simulink model "uz_ssi_interface_2023a"  (R2023a)
settings: Solver=FixedStepDiscrete  StartTime=0.0  StopTime=0.003  RelTol=1e-3
values from neighbouring files (symbols this model uses):
  binary_or_gray = false    [uz_ssi_interface_init.m]
  bit_sum = ssi_encoder_bit_width_multi_turn+ssi_encoder_bit_width_single_turn+ssi_encoder_number_of_status_bits    [uz_ssi_interface_init.m]
  delay_first_clk_on_off = true    [uz_ssi_interface_init.m]
  f_ADC = 10e3    (= 10000)    [uz_ssi_interface_init.m]
  f_clock = 100e6    (= 100000000)    [uz_ssi_interface_init.m]
  ssi_clk_divider = 25    [uz_ssi_interface_init.m]
  ssi_encoder_bit_width_multi_turn = uint32(0)    [uz_ssi_interface_init.m]
  ssi_encoder_bit_width_single_turn = uint32(14)    [uz_ssi_interface_init.m]
  ssi_encoder_number_of_status_bits = uint32(0)    [uz_ssi_interface_init.m]
  t_ADC = 1/f_ADC    (= 0.0001)    [uz_ssi_interface_init.m]
  t_clock = 1/f_clock    (= 1e-08)    [uz_ssi_interface_init.m]
undefined symbols (not defined in the file or in its folder): PLL
libraries: hdlsllib x42, simulink x14, simulink_extras x5, spsSampleandHoldLib x1
(part 1 of 2)
settings Model: DataTypeOverride=Off  Creator=micha  LastModifiedBy=micha
settings SolverCC: AlgebraicLoopSolver=TrustRegion
settings DataIOCC: LimitDataPoints=on  SaveOutput=off  SaveTime=off
settings OptimizationCC: BlockReduction=off  ConditionallyExecuteInputs=off  DefaultParameterBehavior=Inlined  LifeSpan=inf
settings DebuggingCC: AlgebraicLoopMsg=error  SingleTaskRateTransMsg=error  UnconnectedInputMsg=warning  UnconnectedOutputMsg=warning  UnconnectedLineMsg=warning  AllowSymbolicDim=off  StrictBusMsg=ErrorOnBusTreatedAsVector  SFUnexpectedBacktrackingDiag=warning  SFNoUnconditionalDefaultTransitionDiag=warning  SFExecutionAtInitializationDiag=none  ArithmeticOperatorsInVariantConditions=warning
settings HardwareCC: ProdBitPerPointer=32  ProdBitPerSizeT=32  ProdBitPerPtrDiffT=32  ProdLargestAtomicFloat=None  ProdIntDivRoundTo=Undefined  ProdEndianess=Unspecified  ProdWordSize=32  ProdHWDeviceType=ASIC/FPGA->ASIC/FPGA  ProdEqTarget=off
settings ModelReferenceCC: EnableRefExpFcnMdlSchedulingChecks=on
settings SFSimCC: SimUseLocalCustomCode=off  CustomCodeUndefinedFunction=UseInterfaceOnly
settings RTWCC: RTWUseLocalCustomCode=off  DLArmComputeVersion=19.05
settings CodeAppCC: StateflowObjectComments=on
settings GRTTargetCC: TargetLangStandard=C89/C90 (ANSI)
settings ConfigComp: CovScope=ReferencedModels  CovMetricSettings=dw  CovSaveCumulativeToWorkspaceVar=on  CovSaveSingleToWorkspaceVar=on  CovExternalEMLEnable=off  CovSFcnEnable=off

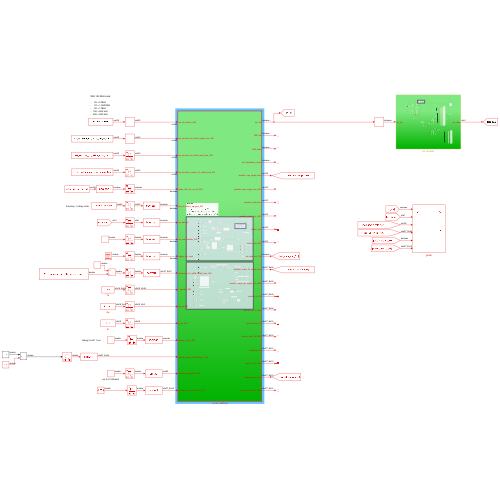
[thumbnail: Simulink's stored preview of the top-level diagram]
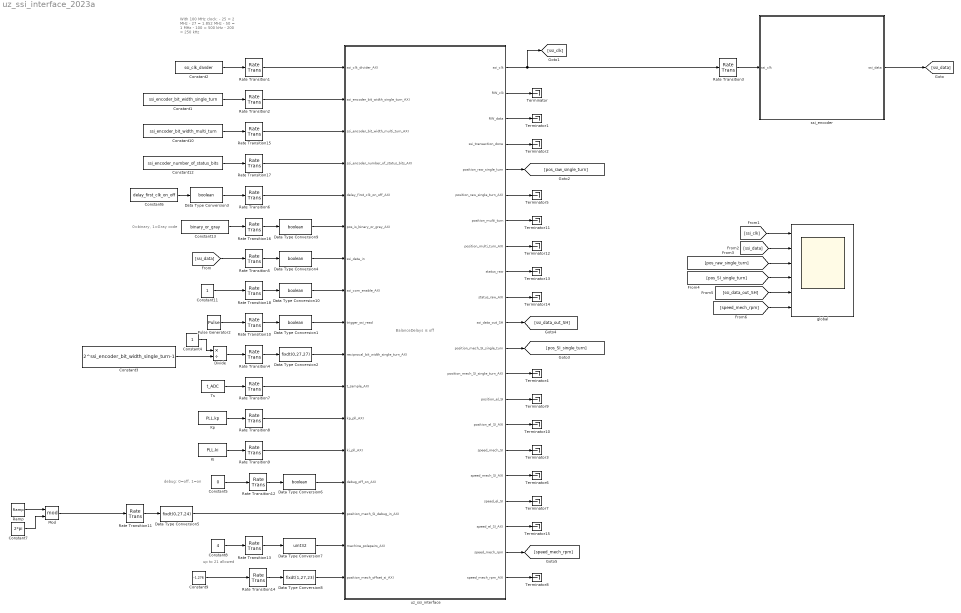
== system uz_ssi_interface_2023a ==
  note: up to 21 allowed
  note: debug: 0=off, 1=on
  note: BalanceDelays is off
  note: With 100 MHz clock:
      |
      | -     25 = 2 MHz
      | -     27 = 1.852 MHz
      | -     50 = 1 MHz
      | -   100 = 500 kHz
      | -   200 = 250 kHz
  note: 0=binary, 1=Gray code
  Constant1 : Constant  Value=ssi_encoder_bit_width_single_turn  OutDataTypeStr=uint32  SampleTime=t_clock
  Constant10 : Constant  Value=ssi_encoder_bit_width_multi_turn  OutDataTypeStr=uint32  SampleTime=t_clock
  Constant11 : Constant  SampleTime=t_clock
  Constant12 : Constant  Value=ssi_encoder_number_of_status_bits  OutDataTypeStr=uint32  SampleTime=t_clock
  Constant13 : Constant  Value=binary_or_gray  OutDataTypeStr=uint32  SampleTime=t_clock
  Constant2 : Constant  Value=ssi_clk_divider  OutDataTypeStr=uint32  SampleTime=t_clock
  Constant3 : Constant  Value=2^ssi_encoder_bit_width_single_turn-1  OutDataTypeStr=double  SampleTime=t_clock
  Constant4 : Constant  SampleTime=t_clock
  Constant5 : Constant  Value=0  SampleTime=t_clock
  Constant6 : Constant  Value=delay_first_clk_on_off  OutDataTypeStr=uint32  SampleTime=t_clock
  Constant7 : Constant  Value=2*pi  SampleTime=t_clock
  Constant8 : Constant  Value=4  SampleTime=t_clock
  Constant9 : Constant  Value=-1.276  SampleTime=t_clock
  Data Type Conversion{1,3..4,6,9..10} (6 alike) : DataTypeConversion  OutDataTypeStr=boolean  SaturateOnIntegerOverflow=off  RndMeth=Floor
  Data Type Conversion2 : DataTypeConversion  OutDataTypeStr=fixdt(0,27,27)  SaturateOnIntegerOverflow=off  RndMeth=Floor
  Data Type Conversion5 : DataTypeConversion  OutDataTypeStr=fixdt(0,27,24)  SaturateOnIntegerOverflow=off  RndMeth=Floor
  Data Type Conversion7 : DataTypeConversion  OutDataTypeStr=uint32  SaturateOnIntegerOverflow=off  RndMeth=Floor
  Data Type Conversion8 : DataTypeConversion  OutDataTypeStr=fixdt(1,27,23)  SaturateOnIntegerOverflow=off  RndMeth=Floor
  Divide : Product  Inputs=*/
  Ki : Constant  Value=PLL.ki  OutDataTypeStr=fixdt(0,18,0)  SampleTime=-1
  Kp : Constant  Value=PLL.kp  OutDataTypeStr=fixdt(0,18,5)  SampleTime=-1
  Mod : Math  Operator=mod
  Pulse Generator2 : DiscretePulseGenerator  Period=f_clock/f_ADC  PulseWidth=0.04*f_clock/f_ADC  SampleTime=t_clock
  Ramp : simulink/Sources/Ramp  slope=2*pi*100  start=7.5e-5  InitialOutput=0
  Rate Transition{1..18} (18 alike) : RateTransition  OutPortSampleTime=t_clock
  Terminator{,1..15} (16 alike) : Terminator
  Ts : Constant  Value=t_ADC  OutDataTypeStr=fixdt(0,18,24)  SampleTime=-1
  global : Scope  NumInputPorts=6
  ssi_encoder : Subsystem
  uz_ssi_interface : Subsystem  TreatAsAtomicUnit=on
  wires:
  Rate Transition10/1 -> Data Type Conversion1/1
  Pulse Generator2/1 -> Rate Transition10/1
  Constant2/1 -> Rate Transition1/1
  Rate Transition1/1 -> uz_ssi_interface/1(ssi_clk_divider_AXI)
  Constant1/1 -> Rate Transition2/1
  Rate Transition2/1 -> uz_ssi_interface/2(ssi_encoder_bit_width_single_turn_AXI)
  Rate Transition3/1 -> ssi_encoder/1(ssi_clk)
  ssi_encoder/1(ssi_data) -> [ssi_data]
  [ssi_data] -> Rate Transition5/1
  uz_ssi_interface/1(ssi_clk) -> [ssi_clk], Rate Transition3/1
  uz_ssi_interface/3(RW_data) -> Terminator1/1
  uz_ssi_interface/4(ssi_transaction_done) -> Terminator2/1
  uz_ssi_interface/2(RW_clk) -> Terminator/1
  Data Type Conversion1/1 -> uz_ssi_interface/9(trigger_ssi_read)
  Rate Transition6/1 -> uz_ssi_interface/5(delay_first_clk_on_off_AXI)
  Data Type Conversion3/1 -> Rate Transition6/1
  Constant6/1 -> Data Type Conversion3/1
  uz_ssi_interface/6(position_raw_single_turn_AXI) -> Terminator5/1
  Rate Transition5/1 -> Data Type Conversion4/1
  Data Type Conversion4/1 -> uz_ssi_interface/7(ssi_data_in)
  Constant3/1 -> Divide/2
  Rate Transition4/1 -> Data Type Conversion2/1
  Data Type Conversion2/1 -> uz_ssi_interface/10(reciprocal_bit_width_single_turn_AXI)
  Constant4/1 -> Divide/1
  Divide/1 -> Rate Transition4/1
  uz_ssi_interface/13(position_mech_SI_single_turn_AXI) -> Terminator4/1
  Ts/1 -> Rate Transition7/1
  Rate Transition7/1 -> uz_ssi_interface/11(t_sample_AXI)
  Kp/1 -> Rate Transition8/1
  Rate Transition8/1 -> uz_ssi_interface/12(kp_pll_AXI)
  Ki/1 -> Rate Transition9/1
  Rate Transition9/1 -> uz_ssi_interface/13(ki_pll_AXI)
  uz_ssi_interface/16(speed_mech_SI) -> Terminator3/1
  uz_ssi_interface/17(speed_mech_SI_AXI) -> Terminator6/1
  Rate Transition11/1 -> Data Type Conversion5/1
  Data Type Conversion5/1 -> uz_ssi_interface/15(position_mech_SI_debug_in_AXI)
  Data Type Conversion6/1 -> uz_ssi_interface/14(debug_off_on_AXI)
  Rate Transition12/1 -> Data Type Conversion6/1
  Constant5/1 -> Rate Transition12/1
  Mod/1 -> Rate Transition11/1
  Ramp/1 -> Mod/1
  Constant7/1 -> Mod/2
  uz_ssi_interface/21(speed_mech_rpm_AXI) -> Terminator8/1
  Rate Transition13/1 -> Data Type Conversion7/1
  Data Type Conversion7/1 -> uz_ssi_interface/16(machine_polepairs_AXI)
  Constant8/1 -> Rate Transition13/1
  Rate Transition14/1 -> Data Type Conversion8/1
  Constant9/1 -> Rate Transition14/1
  Data Type Conversion8/1 -> uz_ssi_interface/17(position_mech_offset_si_AXI)
  uz_ssi_interface/14(position_el_SI) -> Terminator9/1
  uz_ssi_interface/15(position_el_SI_AXI) -> Terminator10/1
  Rate Transition15/1 -> uz_ssi_interface/3(ssi_encoder_bit_width_multi_turn_AXI)
  Constant10/1 -> Rate Transition15/1
  Rate Transition16/1 -> Data Type Conversion9/1
  Constant13/1 -> Rate Transition16/1
  Data Type Conversion9/1 -> uz_ssi_interface/6(pos_is_binary_or_gray_AXI)
  Rate Transition17/1 -> uz_ssi_interface/4(ssi_encoder_number_of_status_bits_AXI)
  Constant12/1 -> Rate Transition17/1
  Data Type Conversion10/1 -> uz_ssi_interface/8(ssi_com_enable_AXI)
  Rate Transition18/1 -> Data Type Conversion10/1
  Constant11/1 -> Rate Transition18/1
  uz_ssi_interface/7(position_multi_turn) -> Terminator11/1
  uz_ssi_interface/8(position_multi_turn_AXI) -> Terminator12/1
  uz_ssi_interface/9(status_raw) -> Terminator13/1
  uz_ssi_interface/10(status_raw_AXI) -> Terminator14/1
  uz_ssi_interface/19(speed_el_SI_AXI) -> Terminator15/1
  uz_ssi_interface/18(speed_el_SI) -> Terminator7/1
  [ssi_clk] -> global/1
  [ssi_data] -> global/2
  uz_ssi_interface/5(position_raw_single_turn) -> [pos_raw_single_turn]
  [pos_raw_single_turn] -> global/3
  [pos_SI_single_turn] -> global/4
  uz_ssi_interface/12(position_mech_SI_single_turn) -> [pos_SI_single_turn]
  uz_ssi_interface/11(ssi_data_out_SH) -> [ssi_data_out_SH]
  [ssi_data_out_SH] -> global/5
  uz_ssi_interface/20(speed_mech_rpm) -> [speed_mech_rpm]
  [speed_mech_rpm] -> global/6

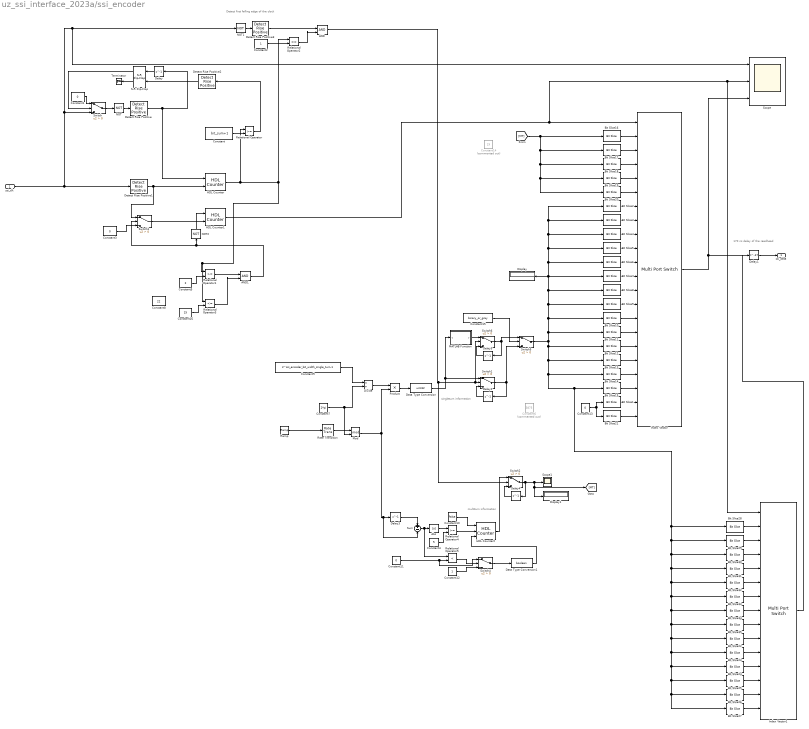
== system uz_ssi_interface_2023a/ssi_encoder ==
  note: multiturn information
  note: 170 ns delay of the readhead
  note: Detect first falling edge of the clock
  note: singleturn information
  ssi_clk : Inport
  AND : Logic  IconShape=distinctive  AllPortsSameDT=off  OutDataTypeStr=boolean
  AND1 : Logic  IconShape=distinctive  AllPortsSameDT=off  OutDataTypeStr=boolean
  Abs : Abs  SaturateOnIntegerOverflow=off
  Bit Slice{1,14,19,26} (4 alike) : hdlsllib/Logic and Bit Operations/Bit Slice  lidx=1  ridx=1
  Bit Slice10 : hdlsllib/Logic and Bit Operations/Bit Slice  lidx=5  ridx=5
  Bit Slice11 : hdlsllib/Logic and Bit Operations/Bit Slice  lidx=4  ridx=4
  Bit Slice12 : hdlsllib/Logic and Bit Operations/Bit Slice  lidx=3  ridx=3
  Bit Slice13 : hdlsllib/Logic and Bit Operations/Bit Slice  lidx=2  ridx=2
  Bit Slice{15,20..21,27} (4 alike) : hdlsllib/Logic and Bit Operations/Bit Slice  lidx=0  ridx=0
  Bit Slice16 : hdlsllib/Logic and Bit Operations/Bit Slice  lidx=4  ridx=4
  Bit Slice17 : hdlsllib/Logic and Bit Operations/Bit Slice  lidx=3  ridx=3
  Bit Slice18 : hdlsllib/Logic and Bit Operations/Bit Slice  lidx=2  ridx=2
  Bit Slice2 : hdlsllib/Logic and Bit Operations/Bit Slice  lidx=13  ridx=13
  Bit Slice22 : hdlsllib/Logic and Bit Operations/Bit Slice  lidx=5  ridx=5
  Bit Slice23 : hdlsllib/Logic and Bit Operations/Bit Slice  lidx=4  ridx=4
  Bit Slice24 : hdlsllib/Logic and Bit Operations/Bit Slice  lidx=3  ridx=3
  Bit Slice25 : hdlsllib/Logic and Bit Operations/Bit Slice  lidx=2  ridx=2
  Bit Slice28 : hdlsllib/Logic and Bit Operations/Bit Slice  lidx=13  ridx=13
  Bit Slice29 : hdlsllib/Logic and Bit Operations/Bit Slice  lidx=12  ridx=12
  Bit Slice3 : hdlsllib/Logic and Bit Operations/Bit Slice  lidx=12  ridx=12
  Bit Slice30 : hdlsllib/Logic and Bit Operations/Bit Slice  lidx=11  ridx=11
  Bit Slice31 : hdlsllib/Logic and Bit Operations/Bit Slice  lidx=10  ridx=10
  Bit Slice32 : hdlsllib/Logic and Bit Operations/Bit Slice  lidx=9  ridx=9
  Bit Slice33 : hdlsllib/Logic and Bit Operations/Bit Slice  lidx=8  ridx=8
  Bit Slice34 : hdlsllib/Logic and Bit Operations/Bit Slice  lidx=7  ridx=7
  Bit Slice35 : hdlsllib/Logic and Bit Operations/Bit Slice  lidx=6  ridx=6
  Bit Slice4 : hdlsllib/Logic and Bit Operations/Bit Slice  lidx=11  ridx=11
  Bit Slice5 : hdlsllib/Logic and Bit Operations/Bit Slice  lidx=10  ridx=10
  Bit Slice6 : hdlsllib/Logic and Bit Operations/Bit Slice  lidx=9  ridx=9
  Bit Slice7 : hdlsllib/Logic and Bit Operations/Bit Slice  lidx=8  ridx=8
  Bit Slice8 : hdlsllib/Logic and Bit Operations/Bit Slice  lidx=7  ridx=7
  Bit Slice9 : hdlsllib/Logic and Bit Operations/Bit Slice  lidx=6  ridx=6
  Constant : Constant  Value=bit_sum+1  SampleTime=t_clock
  Constant1 : Constant  Value=0  SampleTime=t_clock
  Constant10 : Constant  Value=false  SampleTime=t_clock
  Constant11 : Constant  Value=0  SampleTime=t_clock
  Constant12 : Constant  SampleTime=t_clock
  Constant13 : Constant  Value=0  OutDataTypeStr=uint32  SampleTime=t_clock
  Constant14 : Constant  Commented=on  Value=19  OutDataTypeStr=uint32  SampleTime=t_clock
  Constant15 : Constant  Value=binary_or_gray  SampleTime=t_clock
  Constant16 : Constant  Value=15  SampleTime=t_clock
  Constant2 : Constant  SampleTime=t_clock
  Constant3 : Constant  Value=0  OutDataTypeStr=boolean  SampleTime=t_clock
  Constant4 : Constant  Value=5  SampleTime=t_clock
  Constant5 : Constant  Value=2  SampleTime=t_clock
  Constant6 : Constant  Commented=on  Value=3875  OutDataTypeStr=uint32  SampleTime=t_clock
  Constant7 : Constant  Value=2*pi  SampleTime=t_clock
  Constant8 : Constant  Value=22  SampleTime=t_clock
  Constant9 : Constant  Value=2^ssi_encoder_bit_width_single_turn-1  SampleTime=t_clock
  Data Type Conversion : DataTypeConversion  OutDataTypeStr=uint32  SaturateOnIntegerOverflow=off  RndMeth=Floor
  Data Type Conversion1 : DataTypeConversion  OutDataTypeStr=boolean  SaturateOnIntegerOverflow=off  RndMeth=Floor
  Delay : Delay  DelayLength=1
  Delay1 : Delay  DelayLength=17  SampleTime=t_clock
  Delay2 : Delay  DelayLength=1  SampleTime=t_clock
  Delay3 : Delay  DelayLength=1
  Delay4 : Delay  DelayLength=1  InitialCondition=19  SampleTime=t_clock
  Delay5 : Delay  DelayLength=1  SampleTime=t_clock
  Detect Rise Positive{,1..3} (4 alike) : simulink/Logic and Bit Operations/Detect Rise Positive  vinit=0  OutDataTypeStr=boolean
  Display : Display
  Display1 : Display
  Divide : Product  Inputs=*/
  HDL Counter : hdlsllib/Sources/HDL Counter  CountType=Count limited  CountInit=0  CountStep=1  CountMax=bit_sum+1  CountFromType=Initial value  CountFrom=0  CountResetPort=on  CountLoadPort=off  CountEnbPort=on  CountDirPort=off  CountHitOutputPort=off  CountDataType=Unsigned  CountWordLen=8  CountFracLen=0  CountSampTime=t_clock
  HDL Counter1 : hdlsllib/Sources/HDL Counter  CountType=Count limited  CountInit=0  CountStep=1  CountMax=bit_sum+1  CountFromType=Initial value  CountFrom=0  CountResetPort=on  CountLoadPort=off  CountEnbPort=on  CountDirPort=off  CountHitOutputPort=off  CountDataType=Unsigned  CountWordLen=8  CountFracLen=0  CountSampTime=t_clock
  HDL Counter2 : hdlsllib/Sources/HDL Counter  CountType=Count limited  CountInit=19  CountStep=1  CountMax=ssi_encoder_bit_width_multi_turn  CountFromType=Initial value  CountFrom=19  CountResetPort=on  CountLoadPort=off  CountEnbPort=on  CountDirPort=on  CountHitOutputPort=off  CountDataType=Unsigned  CountWordLen=5  CountFracLen=0  CountSampTime=t_clock
  Index Vector : MultiPortSwitch  DataPortOrder=Zero-based contiguous  Inputs=21  zeroidx=on  SaturateOnIntegerOverflow=off  InputSameDT=off
  Index Vector1 : MultiPortSwitch  DataPortOrder=Zero-based contiguous  Inputs=14  zeroidx=on  SaturateOnIntegerOverflow=off  InputSameDT=off
  MATLAB Function : MATLAB Function  TreatAsAtomicUnit=on
  Mod : Math  Operator=mod
  NOT : Logic  Operator=NOT  IconShape=distinctive  AllPortsSameDT=off  OutDataTypeStr=boolean
  NOT1 : Logic  Operator=NOT  IconShape=distinctive  AllPortsSameDT=off  OutDataTypeStr=boolean
  NOT2 : Logic  Operator=NOT  IconShape=distinctive  AllPortsSameDT=off  OutDataTypeStr=boolean
  Product : Product
  Ramp : simulink/Sources/Ramp  slope=-2*pi*50  start=7.5e-5  InitialOutput=0
  Rate Transition : RateTransition  OutPortSampleTime=t_clock
  Relational Operator : RelationalOperator  OutDataTypeStr=boolean  RndMeth=Simplest  InputSameDT=off
  Relational Operator1 : RelationalOperator  OutDataTypeStr=boolean  RndMeth=Simplest  InputSameDT=off
  Relational Operator2 : RelationalOperator  Operator===  OutDataTypeStr=boolean  RndMeth=Simplest  InputSameDT=off
  Relational Operator3 : RelationalOperator  Operator=<=  OutDataTypeStr=boolean  RndMeth=Simplest  InputSameDT=off
  Relational Operator4 : RelationalOperator  OutDataTypeStr=boolean  RndMeth=Simplest  InputSameDT=off
  Relational Operator5 : RelationalOperator  Operator=<  OutDataTypeStr=boolean  RndMeth=Simplest  InputSameDT=off
  S-R Flip-Flop : simulink_extras/Flip Flops/S-R Flip-Flop  initial_condition=0
  Scope : Scope  NumInputPorts=3
  Scope1 : Scope
  Sum : Sum  Inputs=+-
  Switch{,1..6} (7 alike) : Switch  Criteria=u2 > Threshold  SaturateOnIntegerOverflow=off  InputSameDT=off
  Terminator : Terminator
  ssi_data : Outport
  wires:
  NOT/1 -> Detect Rise Positive/1
  Constant/1 -> Relational Operator/2
  Switch/1 -> NOT/1
  S-R Flip-Flop/1 -> Switch/2
  Delay/1 -> S-R Flip-Flop/1
  Relational Operator/1 -> Detect Rise Positive2/1
  Detect Rise Positive2/1 -> S-R Flip-Flop/2
  Detect Rise Positive/1 -> HDL Counter/1, Delay/1
  Relational Operator2/1 -> AND/2
  Constant2/1 -> Relational Operator2/2
  NOT1/1 -> Detect Rise Positive3/1
  Detect Rise Positive3/1 -> AND/1
  Detect Rise Positive1/1 -> HDL Counter/2, Switch3/1
  HDL Counter/1 -> Relational Operator3/1, Relational Operator1/1, Relational Operator2/1, Relational Operator/1
  S-R Flip-Flop/2 -> Terminator/1
  Constant1/1 -> Switch/1
  ssi_clk/1 -> Scope/1, NOT1/1, Switch/3, Detect Rise Positive1/1
  Relational Operator1/1 -> AND1/1
  AND1/1 -> NOT2/1, Switch3/2
  Constant5/1 -> Relational Operator1/2
  Relational Operator3/1 -> AND1/2
  Constant16/1 -> Relational Operator3/2
  Switch3/1 -> HDL Counter1/2
  NOT2/1 -> HDL Counter1/1
  Index Vector/1 -> Scope/3
  Ramp/1 -> Rate Transition/1
  Constant9/1 -> Divide/1
  Divide/1 -> Product/1
  Constant7/1 -> Mod/2, Divide/2
  Product/1 -> Data Type Conversion/1
  Rate Transition/1 -> Mod/1
  Delay2/1 -> Switch1/3
  Data Type Conversion/1 -> Switch1/1, MATLAB Function/1(u)
  AND/1 -> Switch2/2, Switch6/2, Switch1/2
  Constant3/1 -> Switch3/3
  HDL Counter1/1 -> Index Vector1/1, Scope/2, Index Vector/1
  Delay1/1 -> ssi_data/1
  Delay3/1 -> Sum/1
  Mod/1 -> Sum/2, Delay3/1, Product/2
  Sum/1 -> Relational Operator5/1, Abs/1
  Abs/1 -> Relational Operator4/1
  Constant4/1 -> Relational Operator4/2
  Relational Operator4/1 -> HDL Counter2/2
  HDL Counter2/1 -> Switch2/1
  Delay4/1 -> Switch2/3
  Switch2/1 -> [MT], Display1/1, Scope1/1, Delay4/1
  Constant10/1 -> HDL Counter2/1
  Constant11/1 -> Switch4/1, Relational Operator5/2
  Relational Operator5/1 -> Switch4/2
  Switch4/1 -> Data Type Conversion1/1
  Constant12/1 -> Switch4/3
  [MT] -> Bit Slice17/1, Bit Slice18/1, Bit Slice19/1, Bit Slice20/1, Bit Slice16/1
  Bit Slice16/1 -> Index Vector/2
  Bit Slice17/1 -> Index Vector/3
  Bit Slice18/1 -> Index Vector/4
  Bit Slice19/1 -> Index Vector/5
  Bit Slice20/1 -> Index Vector/6
  Bit Slice2/1 -> Index Vector/7
  Bit Slice3/1 -> Index Vector/8
  Bit Slice4/1 -> Index Vector/9
  Bit Slice5/1 -> Index Vector/10
  Bit Slice6/1 -> Index Vector/11
  Bit Slice7/1 -> Index Vector/12
  Bit Slice8/1 -> Index Vector/13
  Bit Slice9/1 -> Index Vector/14
  Bit Slice10/1 -> Index Vector/15
  Bit Slice11/1 -> Index Vector/16
  Bit Slice12/1 -> Index Vector/17
  Bit Slice13/1 -> Index Vector/18
  Bit Slice14/1 -> Index Vector/19
  Bit Slice15/1 -> Index Vector/20
  Bit Slice1/1 -> Index Vector/21
  Bit Slice21/1 -> Index Vector/22
  Constant13/1 -> Bit Slice1/1, Bit Slice21/1
  Data Type Conversion1/1 -> HDL Counter2/3
  Constant15/1 -> Switch5/2
  Switch1/1 -> Delay2/1, Switch5/3
  MATLAB Function/1(y) -> Switch6/1
  Switch6/1 -> Delay5/1, Switch5/1
  Delay5/1 -> Switch6/3
  Switch5/1 -> Bit Slice27/1, Bit Slice26/1, Bit Slice25/1, Bit Slice24/1, Bit Slice23/1, Bit Slice22/1, Bit Slice35/1, Bit Slice34/1, Bit Slice33/1, Bit Slice32/1, Bit Slice31/1, Bit Slice30/1, Bit Slice29/1, Bit Slice28/1, Bit Slice15/1, Bit Slice14/1, Bit Slice13/1, Bit Slice12/1, Display/1, Bit Slice6/1, Bit Slice5/1, Bit Slice4/1, Bit Slice2/1, Bit Slice3/1, Bit Slice7/1, Bit Slice8/1, Bit Slice9/1, Bit Slice10/1, Bit Slice11/1
  Bit Slice29/1 -> Index Vector1/3
  Bit Slice33/1 -> Index Vector1/7
  Bit Slice26/1 -> Index Vector1/14
  Bit Slice22/1 -> Index Vector1/10
  Bit Slice28/1 -> Index Vector1/2
  Bit Slice34/1 -> Index Vector1/8
  Bit Slice23/1 -> Index Vector1/11
  Bit Slice31/1 -> Index Vector1/5
  Bit Slice27/1 -> Index Vector1/15
  Bit Slice35/1 -> Index Vector1/9
  Bit Slice30/1 -> Index Vector1/4
  Bit Slice32/1 -> Index Vector1/6
  Bit Slice25/1 -> Index Vector1/13
  Bit Slice24/1 -> Index Vector1/12
  Index Vector1/1 -> Delay1/1

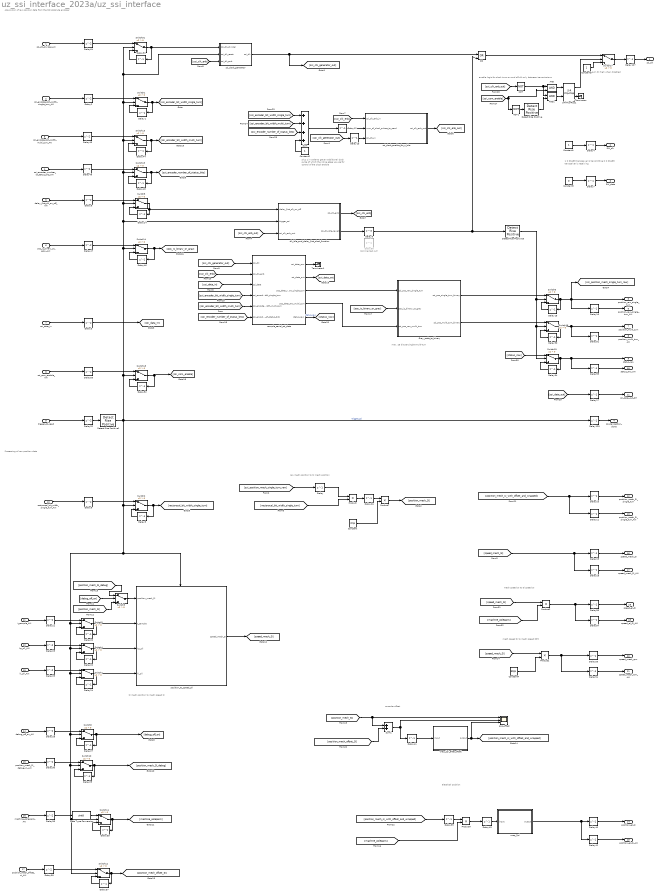
== system uz_ssi_interface_2023a/uz_ssi_interface ==
  note: max. 25 bit per single-/multi-turn
  note: enable logic for clock: turns on and off clk only between transmissions
  note: pull clk high when disabled
  note: plus 1 in order to get an additional clock pulse of which the rising edge we use for control of the clock enable
  note: raw mech position to SI mech position
  note: Processing of raw position data
  note: 1 = RS485 transceiver is transmitting
      | 0 = RS485 transceiver is receiving
  note: Acquisition of raw position data from the SSI absolute encoder
  note: SI mech position to mech speed SI
  note: mech speed SI to mech speed RPM
  note: electrical position
  note: encoder offset
  note: mech speed SI to el speed SI
  ssi_clk_divider_AXI : Inport  OutDataTypeStr=uint32
  ssi_encoder_bit_width_single_turn_AXI : Inport  Port=2  OutDataTypeStr=uint32
  ssi_encoder_bit_width_multi_turn_AXI : Inport  Port=3  OutDataTypeStr=uint32
  ssi_encoder_number_of_status_bits_AXI : Inport  Port=4  OutDataTypeStr=uint32
  delay_first_clk_on_off_AXI : Inport  Port=5  OutDataTypeStr=boolean
  pos_is_binary_or_gray_AXI : Inport  Port=6  OutDataTypeStr=boolean
  ssi_data_in : Inport  Port=7
  ssi_com_enable_AXI : Inport  Port=8  OutDataTypeStr=boolean
  trigger_ssi_read : Inport  Port=9  OutDataTypeStr=boolean
  reciprocal_bit_width_single_turn_AXI : Inport  Port=10
  t_sample_AXI : Inport  Port=11
  kp_pll_AXI : Inport  Port=12
  ki_pll_AXI : Inport  Port=13
  debug_off_on_AXI : Inport  Port=14
  position_mech_SI_debug_in_AXI : Inport  Port=15
  machine_polepairs_AXI : Inport  Port=16
  position_mech_offset_si_AXI : Inport  Port=17
  AND : Logic  IconShape=distinctive  AllPortsSameDT=off  OutDataTypeStr=boolean
  AND1 : Logic  IconShape=distinctive  AllPortsSameDT=off  OutDataTypeStr=boolean
  Constant : Constant  Value=2*pi  OutDataTypeStr=fixdt(0,18,15)  SampleTime=t_clock
  Constant1 : Constant  OutDataTypeStr=boolean  SampleTime=t_clock
  Constant2 : Constant  OutDataTypeStr=uint32  SampleTime=t_clock
  Constant3 : Constant  Value=0  OutDataTypeStr=boolean  SampleTime=t_clock
  Constant4 : Constant  Value=30/pi  OutDataTypeStr=fixdt(0,18,14)  SampleTime=-1
  Constant5 : Constant  OutDataTypeStr=boolean  SampleTime=t_clock
  Data Type Conversion : DataTypeConversion  OutDataTypeStr=uint8  SaturateOnIntegerOverflow=off  RndMeth=Floor
  Delay{,20,22,24,26..27,29,37} (8 alike) : Delay  DelayLength=1  InitialCondition=0
  Delay1 : Delay  DelayLength=1  InitialCondition=ssi_encoder_bit_width_single_turn
  Delay{4,7..8,10..13,16..19,33..34,39..43,56..57,127,129} (22 alike) : Delay  DelayLength=1
  Delay14 : Delay  DelayLength=1  InitialCondition=delay_first_clk_on_off
  Delay{15,50..51,54..55} (5 alike) : Delay  DelayLength=1  InitialCondition=uint32(0)
  Delay{2..3,6,9,21,23,25,28,30,32,36,38,45,47,53,64} (16 alike) : Delay
  Delay31 : Delay  DelayLength=1  InitialCondition=ssi_clk_divider
  Delay35 : Delay  DelayLength=1  InitialCondition=1
  Delay44 : Delay  DelayLength=1  InitialCondition=ssi_encoder_bit_width_multi_turn
  Delay46 : Delay  DelayLength=1  InitialCondition=false
  Delay48 : Delay  DelayLength=1  InitialCondition=uint32(ssi_encoder_number_of_status_bits)
  Delay49 : Delay  InitialCondition=uint32(0)
  Delay5 : Delay  DelayLength=3
  Delay52 : Delay  DelayLength=1  InitialCondition=false
  Delay58 : Delay  Commented=on  DelayLength=1
  Detect Rise Positive : simulink/Logic and Bit Operations/Detect Rise Positive  vinit=0  OutDataTypeStr=boolean
  Detect Rise Positive1 : simulink/Logic and Bit Operations/Detect Rise Positive  vinit=0  OutDataTypeStr=boolean
  Detect Rise Positive3 : simulink/Logic and Bit Operations/Detect Rise Positive  vinit=0  OutDataTypeStr=boolean
  Gray_code_to_binary : Subsystem
  NOT : Logic  Operator=NOT  IconShape=distinctive  AllPortsSameDT=off  OutDataTypeStr=boolean
  NOT1 : Logic  Operator=NOT  IconShape=distinctive  AllPortsSameDT=off  OutDataTypeStr=boolean
  OR : Logic  Operator=OR  IconShape=distinctive  AllPortsSameDT=off  OutDataTypeStr=boolean
  Product : Product  OutDataTypeStr=fixdt(0,27,24)
  Product1 : Product  OutDataTypeStr=fixdt(1,27,12)
  Product2 : Product  OutDataTypeStr=fixdt(1,27,12)
  Product4 : Product  OutDataTypeStr=fixdt(0,27,20)
  Product7 : Product  OutDataTypeStr=fixdt(0,27,24)
  S-R Flip-Flop1 : simulink_extras/Flip Flops/S-R Flip-Flop  initial_condition=0
  Sum : Sum  Inputs=++++  OutDataTypeStr=uint32
  Sum1 : Sum  OutDataTypeStr=fixdt(1,27,23)
  Switch{1..19,31} (20 alike) : Switch  Criteria=u2 > Threshold  SaturateOnIntegerOverflow=off  InputSameDT=off
  Terminator : Terminator
  Terminator1 : Terminator
  clk_idle_and_delay_first_clock_function : Subsystem
  pos_offset : Scope  NumInputPorts=3
  position_to_speed_pll : Subsystem  TreatAsAtomicUnit=on
      settings: LibrarySourceBlock=|
      | hdlsllib/Ports &
      | Subsystems/Triggered
      | Subsystem
  sample_serial_ssi_data : Subsystem
  ssi_clock_enable_for_n_bits : Subsystem
  ssi_clock_generator : Subsystem
  wrap_2pi : Subsystem
  wrap_2pi_after_offset : Subsystem
  ssi_clk : Outport
  RW_clk : Outport  Port=2
  RW_data : Outport  Port=3
  ssi_transaction_done : Outport  Port=4  OutDataTypeStr=boolean  LockScale=on
  position_raw_single_turn : Outport  Port=5  OutDataTypeStr=uint32  LockScale=on
  position_raw_single_turn_AXI : Outport  Port=6  OutDataTypeStr=uint32  LockScale=on
  position_multi_turn : Outport  Port=7  OutDataTypeStr=uint32  LockScale=on
  position_multi_turn_AXI : Outport  Port=8  OutDataTypeStr=uint32  LockScale=on
  status_raw : Outport  Port=9  OutDataTypeStr=uint32  LockScale=on
  status_raw_AXI : Outport  Port=10  OutDataTypeStr=uint32  LockScale=on
  ssi_data_out_SH : Outport  Port=11
  position_mech_SI_single_turn : Outport  Port=12
  position_mech_SI_single_turn_AXI : Outport  Port=13
  position_el_SI : Outport  Port=14
  position_el_SI_AXI : Outport  Port=15
  speed_mech_SI : Outport  Port=16
  speed_mech_SI_AXI : Outport  Port=17
  speed_el_SI : Outport  Port=18
  speed_el_SI_AXI : Outport  Port=19
  speed_mech_rpm : Outport  Port=20
  speed_mech_rpm_AXI : Outport  Port=21
  wires:
  Delay129/1 -> ssi_transaction_done/1
  trigger_ssi_read/1 -> Delay32/1
  Delay32/1 -> Detect Rise Positive1/1
  Delay64/1 -> Switch31/1
  ssi_clk_divider_AXI/1 -> Delay64/1
  Delay31/1 -> Switch31/3
  Switch31/1 -> Delay31/1, ssi_clock_generator/1(ssi_clk_divider)
  Switch1/1 -> Delay1/1, [ssi_encoder_bit_width_single_turn]
  Delay1/1 -> Switch1/3
  ssi_encoder_bit_width_single_turn_AXI/1 -> Delay2/1
  Delay2/1 -> Switch1/1
  ssi_data_in/1 -> Delay3/1
  Delay127/1 -> ssi_clk/1
  [ssi_clk_generator_out] -> Delay13/1
  Delay3/1 -> [ssi_data_in]
  OR/1 -> Switch17/1
  [ssi_data_in] -> sample_serial_ssi_data/3(ssi_data)
  Switch6/1 -> [ssi_position_mech_single_turn_raw], position_raw_single_turn/1, Delay16/1, Delay15/1
  Sum/1 -> Delay12/1
  Delay4/1 -> RW_clk/1
  Delay7/1 -> RW_data/1
  Constant1/1 -> Delay4/1
  Constant3/1 -> Delay7/1
  Switch2/1 -> Delay8/1, [reciprocal_bit_width_single_turn]
  Delay9/1 -> Switch2/1
  Delay8/1 -> Switch2/3
  Delay10/1 -> position_mech_SI_single_turn/1
  Delay11/1 -> position_mech_SI_single_turn_AXI/1
  [ssi_position_mech_single_turn_raw] -> Delay/1
  Delay12/1 -> ssi_clock_enable_for_n_bits/2(num_of_clock_pulses_to_send)
  Delay13/1 -> ssi_clock_enable_for_n_bits/3(ssi_clk_in)
  ssi_clock_enable_for_n_bits/1(ssi_clk_enb_out) -> [ssi_clk_enb_out]
  Constant2/1 -> Sum/4
  [ssi_clk_generator_out] -> sample_serial_ssi_data/1(ssi_clk)
  [ssi_clk_enb] -> ssi_clock_enable_for_n_bits/1(ssi_clk_enb_in)
  delay_first_clk_on_off_AXI/1 -> Delay6/1
  Delay6/1 -> Switch5/1
  Delay14/1 -> Switch5/3
  Switch5/1 -> Delay14/1, clk_idle_and_delay_first_clock_function/1(delay_first_clk_on_off)
  [ssi_clk_enb] -> ssi_clock_generator/3(ssi_clk_enb)
  ssi_clock_generator/1(ssi_clk) -> [ssi_clk_generator_out], OR/1
  Delay15/1 -> Switch6/3
  sample_serial_ssi_data/1(ssi_data_raw) -> Terminator1/1
  Detect Rise Positive3/1 -> Switch6/2, Switch19/2, Switch16/2
  Delay16/1 -> position_raw_single_turn_AXI/1
  clk_idle_and_delay_first_clock_function/2(ssi_clk_idle_levels) -> Delay5/1
  [ssi_clk_enb_out] -> clk_idle_and_delay_first_clock_function/3(ssi_clk_enb_out)
  clk_idle_and_delay_first_clock_function/1(ssi_clk_enb) -> [ssi_clk_enb]
  Delay5/1 -> Detect Rise Positive3/1, OR/2
  [ssi_encoder_bit_width_single_turn] -> sample_serial_ssi_data/4(ssi_encoder_bit_width_single_turn)
  [ssi_clk_enb] -> sample_serial_ssi_data/2(ssi_clk_enb)
  Delay17/1 -> ssi_data_out_SH/1
  sample_serial_ssi_data/2(ssi_data_out) -> [ssi_data_out]
  reciprocal_bit_width_single_turn_AXI/1 -> Delay9/1
  Product/1 -> Delay26/1
  [position_mech_SI] -> Switch9/3
  position_to_speed_pll/1(speed_mech_SI) -> [speed_mech_SI]
  [speed_mech_SI] -> Delay18/1, Delay19/1
  Delay19/1 -> speed_mech_SI/1
  Delay18/1 -> speed_mech_SI_AXI/1
  Delay20/1 -> Switch3/3
  Delay21/1 -> Switch3/1
  Switch3/1 -> position_to_speed_pll/2(t_sample), Delay20/1
  Switch4/1 -> position_to_speed_pll/3(kp_pll), Delay22/1
  Delay23/1 -> Switch4/1
  Delay22/1 -> Switch4/3
  Switch7/1 -> position_to_speed_pll/4(ki_pll), Delay24/1
  Delay25/1 -> Switch7/1
  Delay24/1 -> Switch7/3
  t_sample_AXI/1 -> Delay21/1
  kp_pll_AXI/1 -> Delay23/1
  ki_pll_AXI/1 -> Delay25/1
  Delay/1 -> Product/1
  [reciprocal_bit_width_single_turn] -> Product/2
  Delay26/1 -> Product7/1
  Product7/1 -> [position_mech_SI]
  Switch8/1 -> [debug_off_on], Delay27/1
  Delay28/1 -> Switch8/1
  Delay27/1 -> Switch8/3
  Switch9/1 -> position_to_speed_pll/1(position_mech_SI)
  Delay30/1 -> Switch10/1
  Delay29/1 -> Switch10/3
  Switch10/1 -> [position_mech_SI_debug], Delay29/1
  [debug_off_on] -> Switch9/2
  debug_off_on_AXI/1 -> Delay28/1
  position_mech_SI_debug_in_AXI/1 -> Delay30/1
  [position_mech_SI_debug] -> Switch9/1
  Constant4/1 -> Product1/2
  [speed_mech_SI] -> Product1/1
  Product1/1 -> Delay33/1, Delay34/1
  Delay33/1 -> speed_mech_rpm/1
  Delay34/1 -> speed_mech_rpm_AXI/1
  Delay35/1 -> Switch11/3
  machine_polepairs_AXI/1 -> Delay36/1
  Delay36/1 -> Data Type Conversion/1
  Switch11/1 -> [machine_polepairs], Delay35/1
  Data Type Conversion/1 -> Switch11/1
  Detect Rise Positive1/1 -> Delay129/1, Switch18/2, Switch13/2, Switch31/2, ssi_clock_generator/2(ssi_clk_reset), Switch1/2, Switch15/2, Switch5/2, clk_idle_and_delay_first_clock_function/2(trigger_ssi), Switch14/2, Switch2/2, position_to_speed_pll/Trigger, Switch3/2, Switch4/2, Switch12/2, Switch11/2, Switch10/2, Switch8/2, Switch7/2  "trigger_ssi"
  position_mech_offset_si_AXI/1 -> Delay38/1
  Switch12/1 -> [position_mech_offset_SI], Delay37/1
  Delay38/1 -> Switch12/1
  Delay37/1 -> Switch12/3
  [machine_polepairs] -> Product4/2
  wrap_2pi/1(output) -> Delay42/1, Delay40/1
  [position_mech_si_with_offset_and_wrapped] -> Delay39/1
  Product4/1 -> Delay43/1
  [position_mech_SI] -> pos_offset/1, Sum1/1
  [position_mech_offset_SI] -> Sum1/2
  Sum1/1 -> Delay41/1, pos_offset/2
  wrap_2pi_after_offset/1(output) -> pos_offset/3, [position_mech_si_with_offset_and_wrapped]
  [position_mech_si_with_offset_and_wrapped] -> Delay11/1, Delay10/1
  Delay41/1 -> wrap_2pi_after_offset/1(input)
  Delay39/1 -> Product4/1
  Delay42/1 -> position_el_SI_AXI/1
  Delay40/1 -> position_el_SI/1
  Delay43/1 -> wrap_2pi/1(input)
  Delay44/1 -> Switch13/3
  Switch13/1 -> Delay44/1, [ssi_encoder_bit_width_multi_turn]
  Delay45/1 -> Switch13/1
  ssi_encoder_bit_width_multi_turn_AXI/1 -> Delay45/1
  [ssi_encoder_bit_width_multi_turn] -> sample_serial_ssi_data/5(ssi_encoder_bit_width_multi_turn)
  pos_is_binary_or_gray_AXI/1 -> Delay47/1
  Delay46/1 -> Switch14/3
  Delay47/1 -> Switch14/1
  Switch14/1 -> Delay46/1, [pos_is_binary_or_gray]
  [pos_is_binary_or_gray] -> Gray_code_to_binary/2(pos_is_binary_or_gray)
  Gray_code_to_binary/2(ssi_pos_multi_turn_binary) -> Switch16/1
  Delay49/1 -> Switch15/1
  Switch15/1 -> Delay48/1, [ssi_encoder_number_of_status_bits]
  ssi_encoder_number_of_status_bits_AXI/1 -> Delay49/1
  Delay48/1 -> Switch15/3
  [ssi_encoder_number_of_status_bits] -> sample_serial_ssi_data/6(ssi_encoder_number_of_status_bits)
  [ssi_encoder_bit_width_single_turn] -> Sum/1
  [ssi_encoder_bit_width_multi_turn] -> Sum/2
  [ssi_encoder_number_of_status_bits] -> Sum/3
  sample_serial_ssi_data/4(pos_data_raw_multi_turn) -> Gray_code_to_binary/3(ssi_pos_raw_multi_turn)
  sample_serial_ssi_data/3(pos_data_raw_single_turn) -> Gray_code_to_binary/1(ssi_pos_raw_single_turn)
  Gray_code_to_binary/1(ssi_pos_single_turn_binary) -> Switch6/1
  Switch16/1 -> position_multi_turn/1, Delay51/1, Delay50/1
  Delay51/1 -> position_multi_turn_AXI/1
  Delay50/1 -> Switch16/3
  Constant/1 -> Product7/2
  Switch17/1 -> Delay127/1
  AND/1 -> S-R Flip-Flop1/1
  Constant5/1 -> Switch17/3
  Delay53/1 -> Switch18/1
  ssi_com_enable_AXI/1 -> Delay53/1
  Switch18/1 -> [ssi_com_enable], Delay52/1
  Delay52/1 -> Switch18/3
  [ssi_com_enable] -> AND/2, NOT1/1
  NOT/1 -> AND1/1, AND/1
  [ssi_clk_enb_out] -> NOT/1
  S-R Flip-Flop1/2 -> Terminator/1
  S-R Flip-Flop1/1 -> Switch17/2
  NOT1/1 -> Detect Rise Positive/1
  Detect Rise Positive/1 -> AND1/2
  Delay54/1 -> Switch19/3
  Switch19/1 -> status_raw/1, Delay55/1, Delay54/1
  Delay55/1 -> status_raw_AXI/1
  [ssi_data_out] -> Delay17/1
  [status_raw] -> Switch19/1
  sample_serial_ssi_data/5(status_raw) -> [status_raw]  "status_raw"
  AND1/1 -> S-R Flip-Flop1/2
  [speed_mech_SI] -> Product2/1
  Delay56/1 -> speed_el_SI/1
  Product2/1 -> Delay56/1, Delay57/1
  [machine_polepairs] -> Product2/2
  Delay57/1 -> speed_el_SI_AXI/1

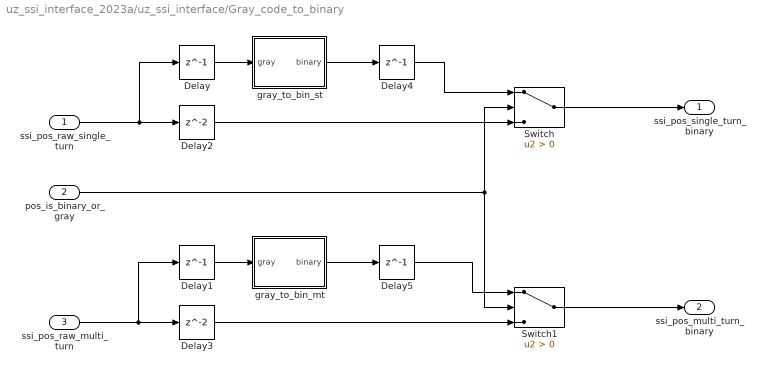
== system uz_ssi_interface_2023a/uz_ssi_interface/Gray_code_to_binary ==
  ssi_pos_raw_single_turn : Inport
  pos_is_binary_or_gray : Inport  Port=2
  ssi_pos_raw_multi_turn : Inport  Port=3
  Delay{,1,4..5} (4 alike) : Delay  DelayLength=1
  Delay2 : Delay
  Delay3 : Delay
  Switch : Switch  Criteria=u2 > Threshold  SaturateOnIntegerOverflow=off  InputSameDT=off
  Switch1 : Switch  Criteria=u2 > Threshold  SaturateOnIntegerOverflow=off  InputSameDT=off
  gray_to_bin_mt : MATLAB Function  TreatAsAtomicUnit=on
  gray_to_bin_st : MATLAB Function  TreatAsAtomicUnit=on
  ssi_pos_single_turn_binary : Outport
  ssi_pos_multi_turn_binary : Outport  Port=2
  wires:
  pos_is_binary_or_gray/1 -> Switch/2, Switch1/2
  Switch/1 -> ssi_pos_single_turn_binary/1
  Switch1/1 -> ssi_pos_multi_turn_binary/1
  gray_to_bin_st/1(binary) -> Delay4/1
  ssi_pos_raw_single_turn/1 -> Delay/1, Delay2/1
  ssi_pos_raw_multi_turn/1 -> Delay1/1, Delay3/1
  gray_to_bin_mt/1(binary) -> Delay5/1
  Delay/1 -> gray_to_bin_st/1(gray)
  Delay1/1 -> gray_to_bin_mt/1(gray)
  Delay2/1 -> Switch/3
  Delay3/1 -> Switch1/3
  Delay4/1 -> Switch/1
  Delay5/1 -> Switch1/1

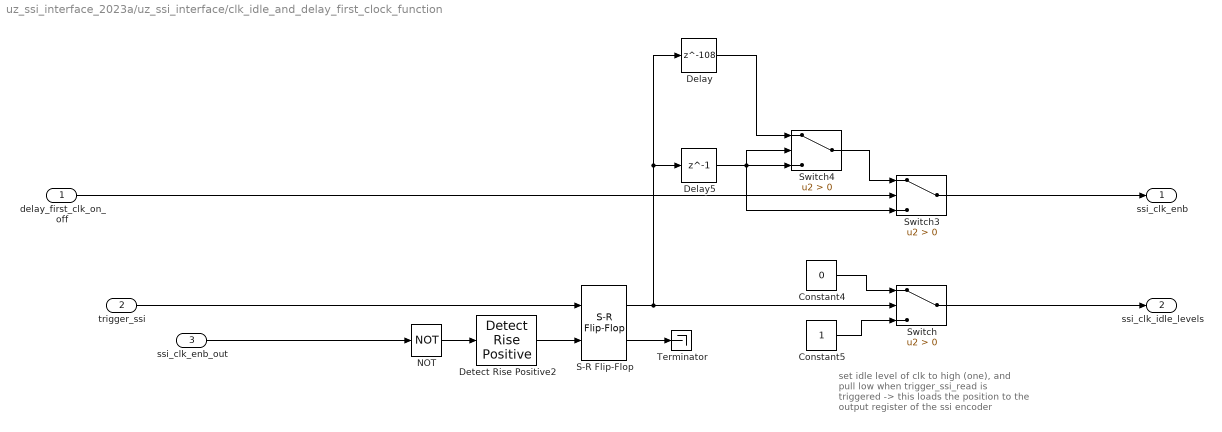
== system uz_ssi_interface_2023a/uz_ssi_interface/clk_idle_and_delay_first_clock_function ==
  note: set idle level of clk to high (one),
      | and pull low when trigger_ssi_read
      | is triggered -> this loads the position to the output register of the ssi encoder
  delay_first_clk_on_off : Inport
  trigger_ssi : Inport  Port=2
  ssi_clk_enb_out : Inport  Port=3
  Constant4 : Constant  Value=0  OutDataTypeStr=boolean  SampleTime=t_clock
  Constant5 : Constant  OutDataTypeStr=boolean  SampleTime=t_clock
  Delay : Delay  DelayLength=108
  Delay5 : Delay  DelayLength=1
  Detect Rise Positive2 : simulink/Logic and Bit Operations/Detect Rise Positive  vinit=0  OutDataTypeStr=boolean
  NOT : Logic  Operator=NOT  IconShape=distinctive  AllPortsSameDT=off  OutDataTypeStr=boolean
  S-R Flip-Flop : simulink_extras/Flip Flops/S-R Flip-Flop  initial_condition=0
  Switch : Switch  Criteria=u2 > Threshold  SaturateOnIntegerOverflow=off  InputSameDT=off
  Switch3 : Switch  Criteria=u2 > Threshold  SaturateOnIntegerOverflow=off  InputSameDT=off
  Switch4 : Switch  Criteria=u2 > Threshold  SaturateOnIntegerOverflow=off  InputSameDT=off
  Terminator : Terminator
  ssi_clk_enb : Outport
  ssi_clk_idle_levels : Outport  Port=2
  wires:
  S-R Flip-Flop/2 -> Terminator/1
  Delay5/1 -> Switch3/3, Switch4/3, Switch4/2
  S-R Flip-Flop/1 -> Switch/2, Delay/1, Delay5/1
  Switch4/1 -> Switch3/1
  Constant5/1 -> Switch/3
  Constant4/1 -> Switch/1
  NOT/1 -> Detect Rise Positive2/1
  Detect Rise Positive2/1 -> S-R Flip-Flop/2
  ssi_clk_enb_out/1 -> NOT/1
  Switch/1 -> ssi_clk_idle_levels/1
  delay_first_clk_on_off/1 -> Switch3/2
  trigger_ssi/1 -> S-R Flip-Flop/1
  Switch3/1 -> ssi_clk_enb/1
  Delay/1 -> Switch4/1

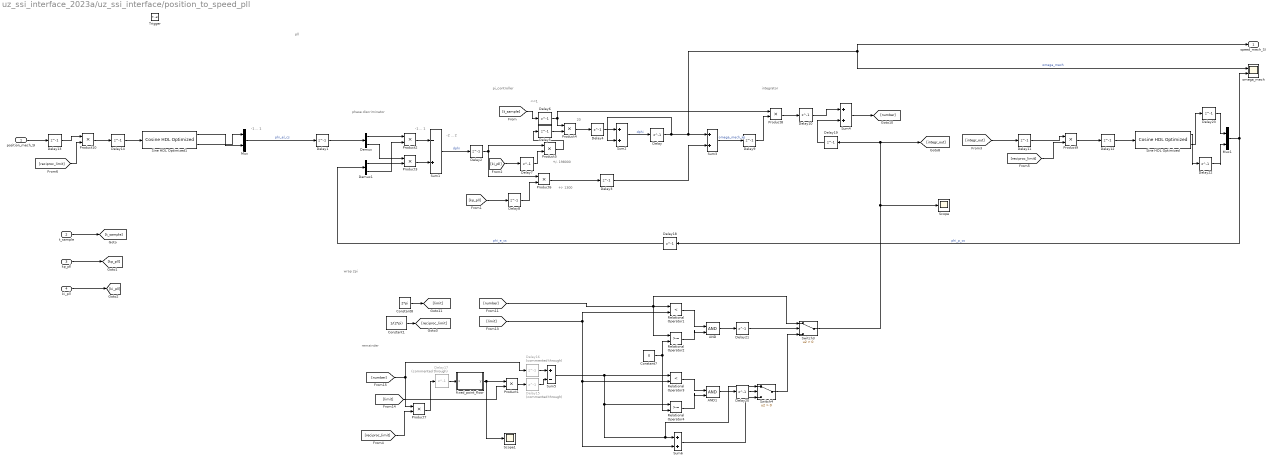
== system uz_ssi_interface_2023a/uz_ssi_interface/position_to_speed_pll ==
  note: remainder
  note: +/- 1300
  note: 20
  note: integrator
  note: -1 ... 1
  note: pll
  note: -1 ... 1
  note: phase discriminator
  note: <<1
  note: wrap 2pi
  note: -2 ... 2
  note: +/- 198000
  note: pi_controller
  position_mech_SI : Inport
  t_sample : Inport  Port=2
  kp_pll : Inport  Port=3
  ki_pll : Inport  Port=4
  Trigger : TriggerPort  VariantControl=(inherit)  InitialTriggerSignalState=zero
  AND : Logic  IconShape=distinctive  AllPortsSameDT=off  OutDataTypeStr=boolean
  AND1 : Logic  IconShape=distinctive  AllPortsSameDT=off  OutDataTypeStr=boolean
  Constant1 : Constant  Value=1/(2*pi)  OutDataTypeStr=fixdt(0,18,20)  SampleTime=-1
  Constant7 : Constant  Value=0  OutDataTypeStr=fixdt(0,27,24)  SampleTime=-1
  Constant8 : Constant  Value=2*pi  OutDataTypeStr=fixdt(0,18,15)  SampleTime=-1
  Delay{,19..23} (6 alike) : Delay  DelayLength=1
  Delay1 : Delay  DelayLength=1  InitialCondition=[1 0]
  Delay{2..14} (13 alike) : Delay  DelayLength=1  InitialCondition=0
  Delay15 : Delay  Commented=through  DelayLength=1  InitialCondition=0
  Delay16 : Delay  Commented=through  DelayLength=1  InitialCondition=0
  Delay17 : Delay  Commented=through  DelayLength=1  InitialCondition=0
  Delay18 : Delay  DelayLength=1  InitialCondition=[1 0]
  Demux : Demux  Outputs=2
  Demux1 : Demux  Outputs=2
  Mux : Mux  Inputs=2
  Mux1 : Mux  Inputs=2
  Product1 : Product  OutDataTypeStr=fixdt(1,27,23)
  Product10 : Product  OutDataTypeStr=fixdt(1,27,20)
  Product2 : Product  OutDataTypeStr=fixdt(1,27,25)
  Product3 : Product  OutDataTypeStr=fixdt(1,27,25)
  Product4 : Product  OutDataTypeStr=fixdt(1,27,20)
  Product5 : Product  OutDataTypeStr=fixdt(1,27,8)
  Product6 : Product  OutDataTypeStr=fixdt(1,27,14)
  Product7 : Product  OutDataTypeStr=fixdt(1,27,23)
  Product8 : Product  OutDataTypeStr=fixdt(1,27,26)
  Product9 : Product  OutDataTypeStr=fixdt(1,27,20)
  Relational Operator1 : RelationalOperator  Operator=<  OutDataTypeStr=boolean  RndMeth=Simplest  InputSameDT=off
  Relational Operator2 : RelationalOperator  OutDataTypeStr=boolean  RndMeth=Simplest  InputSameDT=off
  Relational Operator3 : RelationalOperator  Operator=<  OutDataTypeStr=boolean  RndMeth=Simplest  InputSameDT=off
  Relational Operator4 : RelationalOperator  OutDataTypeStr=boolean  RndMeth=Simplest  InputSameDT=off
  Scope : Scope
  Scope1 : Scope
  Sine HDL Optimized : hdlsllib/Lookup Tables/Cosine HDL Optimized  OutputFormula=sin(2*pi*u) and cos(2*pi*u)  NumDataPoints=256  TableDataTypeStr=fixdt(0,26,20)  SimulateLUTROMDelay=off
      settings: LibrarySourceBlock=|
      | hdlsllib/Lookup
      | Tables/Sine
      | HDL Optimized
  Sine HDL Optimized1 : hdlsllib/Lookup Tables/Cosine HDL Optimized  OutputFormula=sin(2*pi*u) and cos(2*pi*u)  NumDataPoints=256  TableDataTypeStr=fixdt(0,26,20)  SimulateLUTROMDelay=off
      settings: LibrarySourceBlock=|
      | hdlsllib/Lookup
      | Tables/Sine
      | HDL Optimized
  Sum1 : Sum  Inputs=-+  AccumDataTypeStr=fixdt(1,27,24)
  Sum2 : Sum  OutDataTypeStr=fixdt(1,27,16)
  Sum3 : Sum  OutDataTypeStr=fixdt(1,27,14)
  Sum4 : Sum  OutDataTypeStr=fixdt(1,27,23)
  Sum5 : Sum  Inputs=+-  OutDataTypeStr=fixdt(1,27,23)
  Sum6 : Sum  OutDataTypeStr=fixdt(1,27,23)
  Switch3 : Switch  Criteria=u2 > Threshold  SaturateOnIntegerOverflow=off  InputSameDT=off
  Switch4 : Switch  Criteria=u2 > Threshold  SaturateOnIntegerOverflow=off  InputSameDT=off
  fixed_point_floor : MATLAB Function  TreatAsAtomicUnit=on
  omega_mech : Scope  NumInputPorts=2
  speed_mech_SI : Outport  InitialOutput=[0]
  wires:
  Product2/1 -> Sum1/1
  Constant8/1 -> [limit]
  Delay19/1 -> Sum4/2
  Demux/1 -> Product2/1
  Mux1/1 -> omega_mech/2, Delay18/1  "phi_p_cs"
  [ki_pll] -> Delay7/1
  Sine HDL Optimized/2 -> Delay23/1
  Sum3/1 -> Delay9/1  "omega_mech_kp"
  Demux1/2 -> Product2/2
  Switch3/1 -> Scope/1, Delay19/1, [integr_out]
  Product3/1 -> Sum1/2
  Product4/1 -> Delay4/1
  Delay/1 -> speed_mech_SI/1, omega_mech/1, Sum3/1, Sum2/2  "omega_mech"
  Product8/1 -> Delay10/1
  [limit] -> Product1/2
  Switch4/1 -> Switch3/3
  [integr_out] -> Delay11/1
  Product1/1 -> Delay15/1
  Relational Operator3/1 -> AND1/1
  Product9/1 -> Delay12/1
  [number] -> Relational Operator2/1, Switch3/1, Relational Operator1/1
  Relational Operator2/1 -> AND/2
  Sum4/1 -> [number]
  Sum1/1 -> Delay2/1  "dphi"
  [limit] -> Relational Operator1/2, Sum6/2, Relational Operator3/2
  Product5/1 -> Delay5/1
  Product10/1 -> Delay14/1
  [number] -> Product7/1, Delay16/1
  Demux/2 -> Product3/1
  Delay6/1 -> Product4/1, Product8/1
  Demux1/1 -> Product3/2
  Delay18/1 -> Demux1/1  "phi_e_cs"
  Sine HDL Optimized/1 -> Delay22/1
  Mux/1 -> Delay1/1  "phi_el_cs"
  Relational Operator1/1 -> AND/1
  Product6/1 -> Delay3/1
  [kp_pll] -> Delay8/1
  AND/1 -> Delay21/1
  Sine HDL Optimized1/1 -> Mux/2
  Product7/1 -> Delay17/1
  Sum2/1 -> Delay/1  "dphi"
  Sum6/1 -> Switch4/3
  Sine HDL Optimized1/2 -> Mux/1
  Relational Operator4/1 -> AND1/2
  AND1/1 -> Delay20/1
  fixed_point_floor/1(y) -> Product1/1, Scope1/1
  position_mech_SI/1 -> Delay13/1
  Constant7/1 -> Relational Operator2/2, Relational Operator4/2
  t_sample/1 -> [t_sample]
  kp_pll/1 -> [kp_pll]
  ki_pll/1 -> [ki_pll]
  Delay1/1 -> Demux/1
  Delay2/1 -> Product5/1, Product6/1
  Delay3/1 -> Sum3/2
  Delay4/1 -> Sum2/1
  Delay5/1 -> Product4/2
  Delay7/1 -> Product5/2
  Delay8/1 -> Product6/2
  Delay9/1 -> Product8/2
  [t_sample] -> Delay6/1
  Delay10/1 -> Sum4/1
  Delay11/1 -> Product9/1
  Delay12/1 -> Sine HDL Optimized/1
  Delay13/1 -> Product10/1
  Delay14/1 -> Sine HDL Optimized1/1
  Delay15/1 -> Sum5/2
  Delay16/1 -> Sum5/1
  Delay17/1 -> fixed_point_floor/1(x)
  Sum5/1 -> Switch4/1, Sum6/1, Relational Operator4/1, Relational Operator3/1
  Constant1/1 -> [reciproc_limit]
  [reciproc_limit] -> Product7/2
  Delay20/1 -> Switch4/2
  Delay21/1 -> Switch3/2
  [reciproc_limit] -> Product9/2
  [reciproc_limit] -> Product10/2
  Delay22/1 -> Mux1/2
  Delay23/1 -> Mux1/1

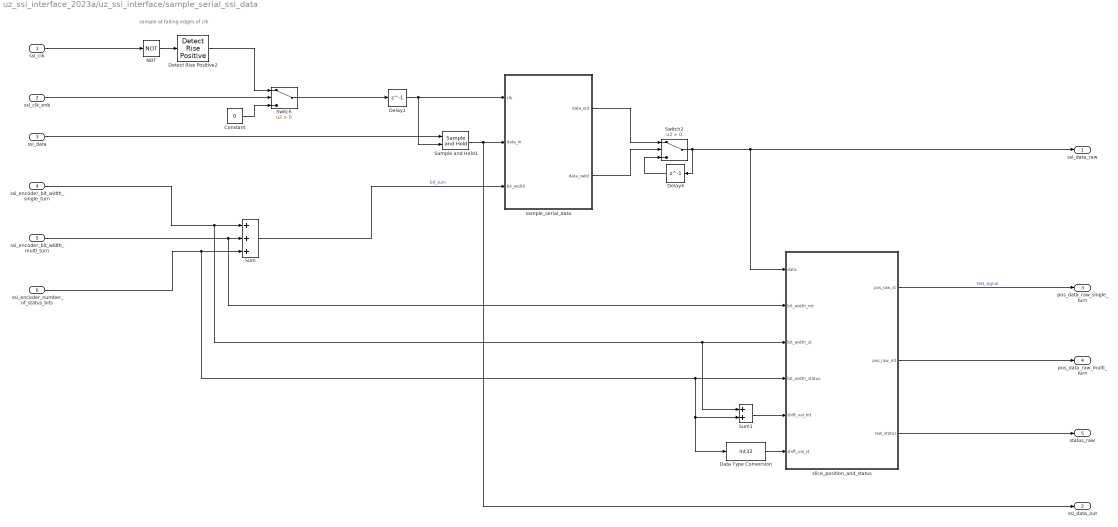
== system uz_ssi_interface_2023a/uz_ssi_interface/sample_serial_ssi_data ==
  note: sample at falling edges of clk
  ssi_clk : Inport
  ssi_clk_enb : Inport  Port=2
  ssi_data : Inport  Port=3
  ssi_encoder_bit_width_single_turn : Inport  Port=4  OutDataTypeStr=uint32
  ssi_encoder_bit_width_multi_turn : Inport  Port=5  OutDataTypeStr=uint32
  ssi_encoder_number_of_status_bits : Inport  Port=6  OutDataTypeStr=uint32
  Constant : Constant  Value=0  OutDataTypeStr=boolean  SampleTime=t_clock
  Data Type Conversion : DataTypeConversion  OutDataTypeStr=int32  SaturateOnIntegerOverflow=off  RndMeth=Floor
  Delay1 : Delay  DelayLength=1  SampleTime=t_clock
  Delay4 : Delay  DelayLength=1  InitialCondition=uint64(0)
  Detect Rise Positive2 : simulink/Logic and Bit Operations/Detect Rise Positive  vinit=0  OutDataTypeStr=boolean
  NOT : Logic  Operator=NOT  IconShape=distinctive  AllPortsSameDT=off  OutDataTypeStr=boolean
  Sample and Hold1 : spsSampleandHoldLib/Sample and Hold  ic=0  Ts=t_clock
      settings: LibrarySourceBlock=|
      | sps_lib/Control/Sample and
      | Hold
  Sum : Sum  Inputs=+++  OutDataTypeStr=uint32
  Sum1 : Sum  OutDataTypeStr=int32
  Switch : Switch  Criteria=u2 > Threshold  SaturateOnIntegerOverflow=off  InputSameDT=off
  Switch2 : Switch  Criteria=u2 > Threshold  SaturateOnIntegerOverflow=off  InputSameDT=off
  sample_serial_data : MATLAB Function  TreatAsAtomicUnit=on
  slice_position_and_status : MATLAB Function  TreatAsAtomicUnit=on
  ssi_data_raw : Outport  OutDataTypeStr=uint64
  ssi_data_out : Outport  Port=2
  pos_data_raw_single_turn : Outport  Port=3
  pos_data_raw_multi_turn : Outport  Port=4
  status_raw : Outport  Port=5
  wires:
  Delay4/1 -> Switch2/3
  ssi_encoder_bit_width_single_turn/1 -> Sum1/1, slice_position_and_status/3(bit_width_st), Sum/1
  Detect Rise Positive2/1 -> Switch/1
  Delay1/1 -> Sample and Hold1/2, sample_serial_data/1(clk)
  NOT/1 -> Detect Rise Positive2/1
  ssi_data/1 -> Sample and Hold1/1
  ssi_clk_enb/1 -> Switch/2
  Switch/1 -> Delay1/1
  Constant/1 -> Switch/3
  sample_serial_data/1(data_out) -> Switch2/1
  sample_serial_data/2(data_valid) -> Switch2/2
  Sample and Hold1/1 -> ssi_data_out/1, sample_serial_data/2(data_in)
  ssi_clk/1 -> NOT/1
  Sum/1 -> sample_serial_data/3(bit_width)  "bit_sum"
  ssi_encoder_bit_width_multi_turn/1 -> slice_position_and_status/2(bit_width_mt), Sum/2
  slice_position_and_status/3(raw_status) -> status_raw/1
  slice_position_and_status/2(pos_raw_mt) -> pos_data_raw_multi_turn/1
  Switch2/1 -> ssi_data_raw/1, slice_position_and_status/1(data), Delay4/1
  Sum1/1 -> slice_position_and_status/5(shift_val_mt)
  ssi_encoder_number_of_status_bits/1 -> Data Type Conversion/1, Sum1/2, slice_position_and_status/4(bit_width_status), Sum/3
  Data Type Conversion/1 -> slice_position_and_status/6(shift_val_st)
  slice_position_and_status/1(pos_raw_st) -> pos_data_raw_single_turn/1  "test_signal"

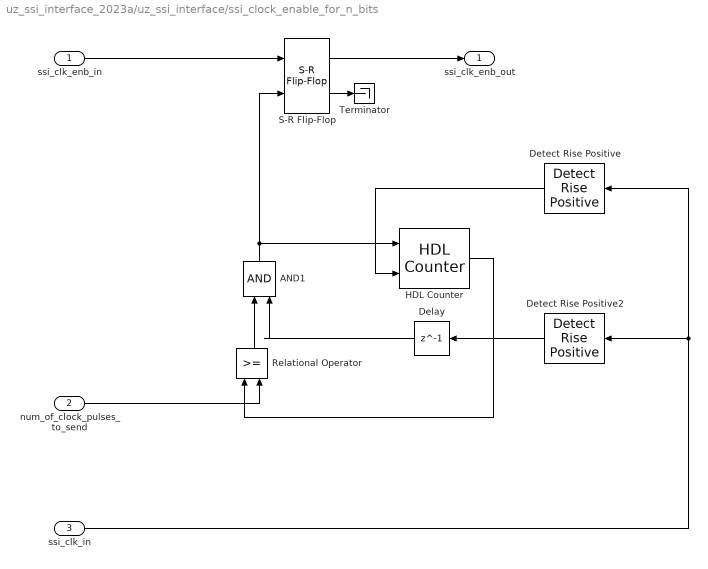
== system uz_ssi_interface_2023a/uz_ssi_interface/ssi_clock_enable_for_n_bits ==
  ssi_clk_enb_in : Inport
  num_of_clock_pulses_to_send : Inport  Port=2
  ssi_clk_in : Inport  Port=3
  AND1 : Logic  IconShape=distinctive  AllPortsSameDT=off  OutDataTypeStr=boolean
  Delay : Delay  DelayLength=1
  Detect Rise Positive : simulink/Logic and Bit Operations/Detect Rise Positive  vinit=0  OutDataTypeStr=boolean
  Detect Rise Positive2 : simulink/Logic and Bit Operations/Detect Rise Positive  vinit=0  OutDataTypeStr=boolean
  HDL Counter : hdlsllib/Sources/HDL Counter  CountType=Free running  CountInit=0  CountStep=1  CountMax=25  CountFromType=Initial value  CountFrom=0  CountResetPort=on  CountLoadPort=off  CountEnbPort=on  CountDirPort=off  CountHitOutputPort=off  CountDataType=Unsigned  CountWordLen=8  CountFracLen=0  CountSampTime=1
  Relational Operator : RelationalOperator  OutDataTypeStr=boolean  RndMeth=Simplest  InputSameDT=off
  S-R Flip-Flop : simulink_extras/Flip Flops/S-R Flip-Flop  initial_condition=0
  Terminator : Terminator
  ssi_clk_enb_out : Outport
  wires:
  HDL Counter/1 -> Relational Operator/1
  num_of_clock_pulses_to_send/1 -> Relational Operator/2
  Detect Rise Positive2/1 -> Delay/1
  S-R Flip-Flop/2 -> Terminator/1
  Relational Operator/1 -> AND1/1
  Detect Rise Positive/1 -> HDL Counter/2
  AND1/1 -> HDL Counter/1, S-R Flip-Flop/2
  ssi_clk_in/1 -> Detect Rise Positive2/1, Detect Rise Positive/1
  S-R Flip-Flop/1 -> ssi_clk_enb_out/1
  Delay/1 -> AND1/2
  ssi_clk_enb_in/1 -> S-R Flip-Flop/1

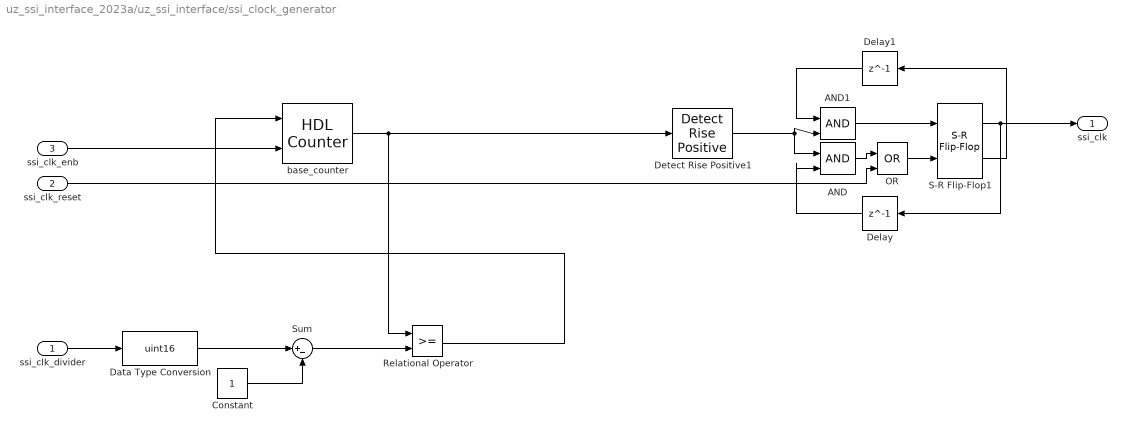
== system uz_ssi_interface_2023a/uz_ssi_interface/ssi_clock_generator ==
  ssi_clk_divider : Inport
  ssi_clk_reset : Inport  Port=2
  ssi_clk_enb : Inport  Port=3
  AND : Logic  IconShape=distinctive  AllPortsSameDT=off  OutDataTypeStr=boolean
  AND1 : Logic  IconShape=distinctive  AllPortsSameDT=off  OutDataTypeStr=boolean
  Constant : Constant  OutDataTypeStr=uint16  SampleTime=t_clock
  Data Type Conversion : DataTypeConversion  OutDataTypeStr=uint16  SaturateOnIntegerOverflow=off  RndMeth=Floor
  Delay : Delay  DelayLength=1
  Delay1 : Delay  DelayLength=1
  Detect Rise Positive1 : simulink/Logic and Bit Operations/Detect Rise Positive  vinit=0  OutDataTypeStr=boolean
  OR : Logic  Operator=OR  IconShape=distinctive  AllPortsSameDT=off  OutDataTypeStr=boolean
  Relational Operator : RelationalOperator  OutDataTypeStr=boolean  RndMeth=Simplest  InputSameDT=off
  S-R Flip-Flop1 : simulink_extras/Flip Flops/S-R Flip-Flop  initial_condition=0
  Sum : Sum  Inputs=|+-  AccumDataTypeStr=uint16
  base_counter : hdlsllib/Sources/HDL Counter  CountType=Free running  CountInit=0  CountStep=1  CountMax=199  CountFromType=Initial value  CountFrom=0  CountResetPort=on  CountLoadPort=off  CountEnbPort=on  CountDirPort=off  CountHitOutputPort=off  CountDataType=Unsigned  CountWordLen=16  CountFracLen=0  CountSampTime=1
  ssi_clk : Outport
  wires:
  base_counter/1 -> Relational Operator/1, Detect Rise Positive1/1
  ssi_clk_reset/1 -> OR/2
  Detect Rise Positive1/1 -> AND/1, AND1/2
  S-R Flip-Flop1/1 -> ssi_clk/1, Delay/1
  S-R Flip-Flop1/2 -> Delay1/1
  Delay/1 -> AND/2
  Delay1/1 -> AND1/1
  AND/1 -> OR/1
  ssi_clk_divider/1 -> Data Type Conversion/1
  Data Type Conversion/1 -> Sum/1
  Constant/1 -> Sum/2
  Sum/1 -> Relational Operator/2
  Relational Operator/1 -> base_counter/1
  AND1/1 -> S-R Flip-Flop1/1
  OR/1 -> S-R Flip-Flop1/2
  ssi_clk_enb/1 -> base_counter/2
